simulink model "EKF2017a"  (R2017a)
settings: Solver=VariableStepAuto  StartTime=0.0  StopTime=inf  FixedStep=10e-3  RelTol=1e-3
values from neighbouring files (symbols this model uses):
  imu = rossubscriber('/imu')    [identification.m]
undefined symbols (not defined in the file or in its folder): Angular, Linear
libraries: robotlib x3, sharedTrackingLibrary x1, commseqgen3 x1, etargetslib x1, dspnetwork x1, simulink x1
settings Model: Creator=alic  LastModifiedBy=alic

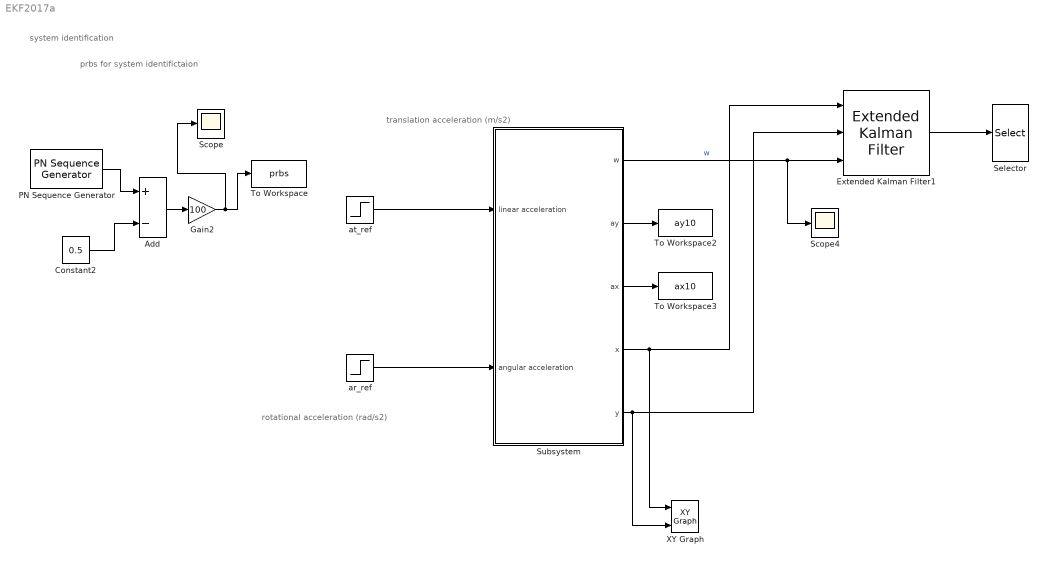
== system EKF2017a ==
  note: prbs for system
      | identifictaion
  note: rotational acceleration
      | (rad/s2)
  note: translation acceleration
      | (m/s2)
  note: system identification
  Add : Sum  Inputs=+-
  Constant2 : Constant  Value=0.5
  Extended Kalman Filter1 : sharedTrackingLibrary/Extended Kalman Filter  StateTransitionFcn=myStateTransitionFcn  HasStateTransitionJacobianFcn=off  HasAdditiveProcessNoise=Additive  ProcessNoise=1  HasTimeVaryingProcessNoise=off  HasStateTransitionFcnExtraArgument=0  InitialState=0  InitialStateCovariance=1  MeasurementFcn1=myMeasurementFcn  HasMeasurementJacobianFcn1=off  HasMeasurementEnablePort1=off  HasAdditiveMeasurementNoise1=Additive  MeasurementNoise1=1  HasTimeVaryingMeasurementNoise1=off  HasMeasurementFcnExtraArgument1=0  MeasurementFcn2=myMeasurementFcn  HasMeasurementJacobianFcn2=off  HasMeasurementEnablePort2=off  HasAdditiveMeasurementNoise2=Nonadditive  MeasurementNoise2=1  HasTimeVaryingMeasurementNoise2=off  HasMeasurementFcnExtraArgument2=0  MeasurementFcn3=myMeasurementFcn  HasMeasurementJacobianFcn3=off  HasMeasurementEnablePort3=off  HasAdditiveMeasurementNoise3=Additive  MeasurementNoise3=1  HasTimeVaryingMeasurementNoise3=off  HasMeasurementFcnExtraArgument3=0  MeasurementFcn4=myMeasurementFcn  HasMeasurementJacobianFcn4=off  HasMeasurementEnablePort4=off  HasAdditiveMeasurementNoise4=Additive  MeasurementNoise4=1  HasTimeVaryingMeasurementNoise4=off  HasMeasurementFcnExtraArgument4=0  MeasurementFcn5=myMeasurementFcn  HasMeasurementJacobianFcn5=off  HasMeasurementEnablePort5=off  HasAdditiveMeasurementNoise5=Additive  MeasurementNoise5=1  HasTimeVaryingMeasurementNoise5=off  HasMeasurementFcnExtraArgument5=0  EnableMultirate=off  StateTransitionFcnSampleTime=1  MeasurementFcn1SampleTime=1  MeasurementFcn2SampleTime=1  MeasurementFcn3SampleTime=1  MeasurementFcn4SampleTime=1  MeasurementFcn5SampleTime=1  UseCurrentEstimator=on  OutputStateCovariance=off  DataType=double  SampleTime=1  NumberOfMeasurements=3
      settings: SourceProductName=Control System Toolbox  SourceProductBaseCode=CT
  Gain2 : Gain  Gain=100
  PN Sequence Generator : commseqgen3/PN Sequence Generator  poly='z^8 + z^6 + z^5 + z^4 + 1'  ini_sta=[0 0 0 0 0 0 0 1]  outBitMaskSource=Dialog parameter  shift=0  outVarSiz=off  maxOutSizeMode=Dialog parameter  maxOutSize=[10 1]  Ts=-1  sampPerFrame=1  reset=off  bitPackedOutputs=off  outDataType=double  numPackedBits=8  bitPackDataSigned=off  bitPackedOutDType=double
      settings: SourceProductName=Communications System Toolbox
  Scope : Scope
  Scope4 : Scope
  Selector : Selector  InputPortWidth=6  IndexOptions=Index vector (dialog)  Indices=[1]  OutputSizes=1
  Subsystem : Subsystem
  To Workspace : ToWorkspace  VariableName=prbs  SaveFormat=Timeseries  SampleTime=-1
  To Workspace2 : ToWorkspace  VariableName=ay10  SaveFormat=Timeseries  SampleTime=-1
  To Workspace3 : ToWorkspace  VariableName=ax10  SaveFormat=Timeseries  SampleTime=-1
  XY Graph : simulink/Sinks/XY Graph  xmin=0  xmax=2000  ymin=0  ymax=1300  st=-1
  ar_ref : Step  Time=0  After=0.9  SampleTime=0
  at_ref : Step  Time=0  After=0.9  SampleTime=0
  wires:
  Subsystem/1(w) -> Scope4/1, Extended Kalman Filter1/3  "w"
  Constant2/1 -> Add/2
  PN Sequence Generator/1 -> Add/1
  Add/1 -> Gain2/1
  Gain2/1 -> Scope/1, To Workspace/1
  Subsystem/2(ay) -> To Workspace2/1
  Subsystem/3(ax) -> To Workspace3/1
  Extended Kalman Filter1/1 -> Selector/1
  at_ref/1 -> Subsystem/1(linear acceleration)
  ar_ref/1 -> Subsystem/2(angular acceleration)
  Subsystem/5(y) -> XY Graph/2, Extended Kalman Filter1/2
  Subsystem/4("x ") -> Extended Kalman Filter1/1, XY Graph/1

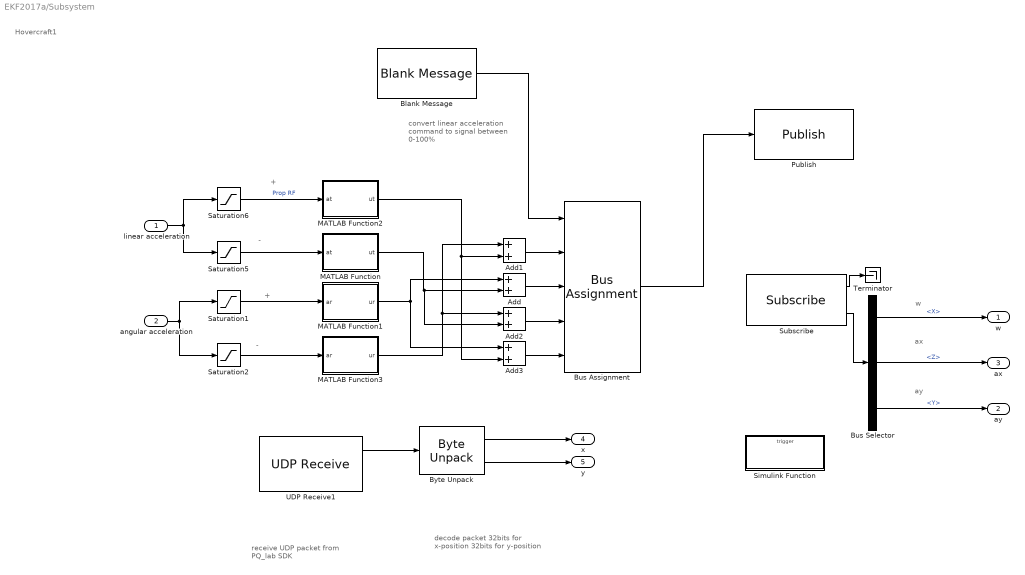
== system EKF2017a/Subsystem ==
  note: convert linear
      | acceleration command
      | to signal between 0-100%
  note: receive UDP packet
      | from PQ_lab SDK
  note: decode packet
      | 32bits for x-position
      | 32bits for y-position
  note: -
  note: +
  note: -
  note: +
  note: Hovercraft1
  note: ay
  note: w
  note: ax
  linear acceleration : Inport
  angular acceleration : Inport  Port=2
  Add{,1..3} (4 alike) : Sum
  Blank Message : robotlib/Blank Message  SourceLibraryInfo=This block requires Robotics System Toolbox  messageType=geometry_msgs/Twist  SampleTime=inf
      settings: SourceProductBaseCode=RO
  Bus Assignment : BusAssignment  AssignedSignals=Linear.X,Linear.Y,Angular.X,Angular.Y
  Bus Selector : BusSelector  OutputSignals=AngularVelocity.X,LinearAcceleration.Z,LinearAcceleration.Y
  Byte Unpack : etargetslib/Byte Unpack  dimensions={[1], [1]}  datatypes={'uint32', 'uint32'}  byteAlign=1
  MATLAB Function : MATLAB Function  TreatAsAtomicUnit=on
  MATLAB Function1 : MATLAB Function  TreatAsAtomicUnit=on
  MATLAB Function2 : MATLAB Function  TreatAsAtomicUnit=on
  MATLAB Function3 : MATLAB Function  TreatAsAtomicUnit=on
  Publish : robotlib/Publish  SourceLibraryInfo=This block requires Robotics System Toolbox  topicSource=Select from ROS network  topic=/cmd_vel  messageType=geometry_msgs/Twist  messageQueueLength=1
      settings: SourceProductBaseCode=RO
  Saturation1 : Saturate  UpperLimit=inf  LowerLimit=0
  Saturation2 : Saturate  UpperLimit=0  LowerLimit=-inf
  Saturation5 : Saturate  UpperLimit=0  LowerLimit=-inf
  Saturation6 : Saturate  UpperLimit=inf  LowerLimit=0
  Simulink Function : Subsystem  TreatAsAtomicUnit=on
  Subscribe : robotlib/Subscribe  SourceLibraryInfo=This block requires Robotics System Toolbox  topicSource=Select from ROS network  topic=/imu  messageType=sensor_msgs/Imu  sampleTime=-1  messageQueueLength=1
      settings: SourceProductBaseCode=RO
  Terminator : Terminator
  UDP Receive1 : dspnetwork/UDP Receive  localURL='0.0.0.0'  localPort=10115  remoteURL='0.0.0.0'  remotePort=-1  recvBufferSize=8192  dims=8  signalDatatype=uint8  isVarSize=off  showBlockingTime=off  blockingTime=0  sampletime=0.1  blockPlatform=[]
      settings: SourceProductName=DSP System Toolbox  SourceProductBaseCode=DS
  w : Outport
  ay : Outport  Port=2
  ax : Outport  Port=3
  "x " : Outport  Port=4
  y : Outport  Port=5
  wires:
  Bus Assignment/1 -> Publish/1
  Subscribe/1 -> Terminator/1
  Subscribe/2 -> Bus Selector/1
  Bus Selector/3 -> ay/1  "<Y>"
  Bus Selector/2 -> ax/1  "<Z>"
  Bus Selector/1 -> w/1  "<X>"
  Blank Message/1 -> Bus Assignment/1
  linear acceleration/1 -> Saturation5/1, Saturation6/1
  Saturation5/1 -> MATLAB Function/1(at)
  Saturation6/1 -> MATLAB Function2/1(at)  "Prop RF"
  angular acceleration/1 -> Saturation1/1, Saturation2/1
  Saturation1/1 -> MATLAB Function1/1(ar)
  Saturation2/1 -> MATLAB Function3/1(ar)
  Add1/1 -> Bus Assignment/2
  Add/1 -> Bus Assignment/3
  Add2/1 -> Bus Assignment/4
  Add3/1 -> Bus Assignment/5
  MATLAB Function3/1(ur) -> Add2/1, Add1/1
  MATLAB Function1/1(ur) -> Add3/1, Add/1
  MATLAB Function2/1(ut) -> Add1/2, Add3/2
  MATLAB Function/1(ut) -> Add2/2, Add/2
  UDP Receive1/1 -> Byte Unpack/1
  Byte Unpack/1 -> "x "/1
  Byte Unpack/2 -> y/1

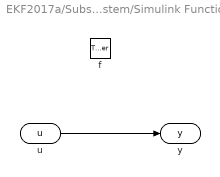
== system EKF2017a/Subsystem/Simulink Function ==
  f : TriggerPort  TriggerType=function-call  IsSimulinkFunction=on  FunctionName=f  VariantControl=(inherit)
  u : ArgIn  DisableCoverage=on  ArgumentName=u
  y : ArgOut  DisableCoverage=on  ArgumentName=y
  wires:
  u/1 -> y/1

== matlab function EKF2017a/Subsystem/MATLAB Function1 ==
  data: ar input; ur output
function ur = fr(ar)
    % we values were really identified
    ur = interp1([0, 6.3632, 16.8374, 25.6822, 35.5810, 45.7588, 53.0103, 60.5996, 83.5957, 89.0708, 96.1055],0:10:100,ar);
end

== matlab function EKF2017a/Subsystem/MATLAB Function ==
  data: at input; ut output
function ut = ft(at)
% values not identified. We just added a -1 to  the one for the positive
% translation
ut=-interp1q([0,0.2244,0.3850,0.6309,0.7839,1.022,1.1630,1.3959,1.5340],[0,2,3,5,6,7,8,9,10],at);
end

== matlab function EKF2017a/Subsystem/MATLAB Function2 ==
  data: at input; ut output
function ut = ft(at)
% these values were really identified
ut=interp1q([0,0.2244,0.3850,0.6309,0.7839,1.022,1.1630,1.3959,1.5340],[0,2,3,5,6,7,8,9,10],at);
end

== matlab function EKF2017a/Subsystem/MATLAB Function3 ==
  data: ar input; ur output
function ur = fr(ar)
% values not identified. We just added a -1 to  the one for the positive rotation
ur = -interp1([0, 6.3632, 16.8374, 25.6822, 35.5810, 45.7588, 53.0103, 60.5996, 83.5957, 89.0708, 96.1055],0:10:100,ar);
end
